simulink model "sy2_08022311"  (R2022b)
settings: Solver=VariableStepAuto  StartTime=0.0  StopTime=20  RelTol=1e-3
settings Model: Creator=赵晨琨  LastModifiedBy=ASUS
settings SolverCC: AlgebraicLoopSolver=TrustRegion
settings DataIOCC: Refine=3
settings DebuggingCC: UnconnectedInputMsg=warning  UnconnectedOutputMsg=warning  UnconnectedLineMsg=warning  SFMachineParentedDataDiag=warning
settings ModelReferenceCC: EnableRefExpFcnMdlSchedulingChecks=on

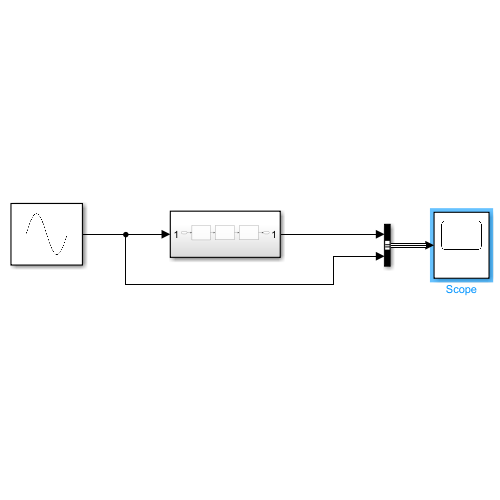
[thumbnail: Simulink's stored preview of the top-level diagram]
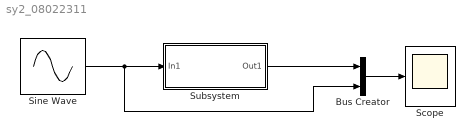
== system sy2_08022311 ==
  Bus Creator : BusCreator  Inputs=2
  Scope : Scope
  Sine Wave : Sin  Phase=1  SampleTime=0
  Subsystem : Subsystem
  wires:
  Sine Wave/1 -> Bus Creator/2, Subsystem/1(In1)
  Subsystem/1(Out1) -> Bus Creator/1
  Bus Creator/1 -> Scope/1

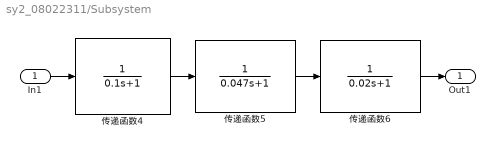
== system sy2_08022311/Subsystem ==
  In1 : Inport
  传递函数4 : TransferFcn  Denominator=[0.1 1]
  传递函数5 : TransferFcn  Denominator=[0.047 1]
  传递函数6 : TransferFcn  Denominator=[0.02 1]
  Out1 : Outport
  wires:
  传递函数4/1 -> 传递函数5/1
  传递函数5/1 -> 传递函数6/1
  传递函数6/1 -> Out1/1
  In1/1 -> 传递函数4/1
